simulink model "new_non_linear"  (R2022b)
settings: Solver=VariableStepAuto  StartTime=0.0  StopTime=10.0  RelTol=1e-3
values from neighbouring files (symbols this model uses):
  e_AG = 0.2    [constantes_NoLineal.m]
  e_AN = 0.2    [constantes_NoLineal.m]
  e_GA = 1-e_AG    (= 0.8)    [constantes_NoLineal.m]
  e_GP = 0.7    [constantes_NoLineal.m]
  e_NA = 1-e_AN    (= 0.8)    [constantes_NoLineal.m]
  e_NP = 0.7    [constantes_NoLineal.m]
  pob_a = 50000    [constantes_NoLineal.m]
  pob_g = 30000    [constantes_NoLineal.m]
  pob_n = 30000    [constantes_NoLineal.m]
  pob_p = 50000    [constantes_NoLineal.m]
  rc_a = 0.003    [constantes_NoLineal.m]
  rc_g = 0.8    [constantes_NoLineal.m]
  rc_n = 0.8    [constantes_NoLineal.m]
  rc_p = 0.003    [constantes_NoLineal.m]
  scale = 1    [constantes_NoLineal.m]
  T_a = 0.2    [constantes_NoLineal.m]
  T_g = 0.7    [constantes_NoLineal.m]
  T_n = 0.7    [constantes_NoLineal.m]
  T_p = 0.2    [constantes_NoLineal.m]
settings Model: Creator=mluser  LastModifiedBy=Hoyos O

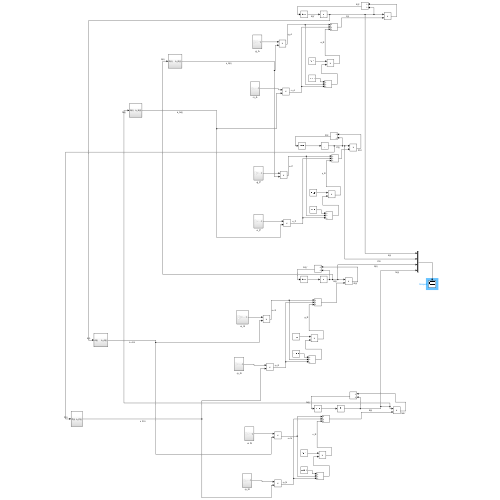
[thumbnail: Simulink's stored preview of the top-level diagram]
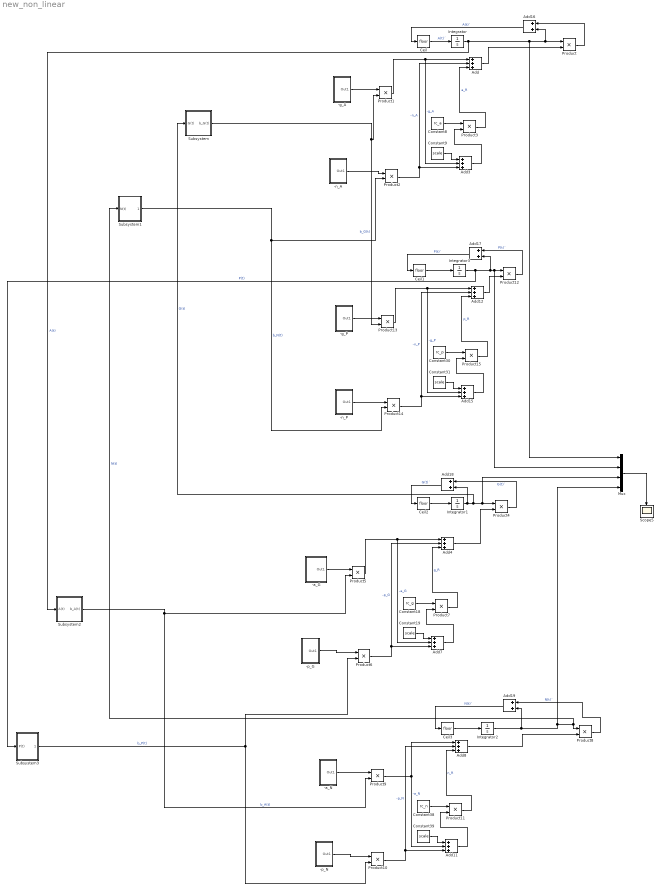
== system new_non_linear ==
  -a_G : Subsystem
  -a_N : Subsystem
  -g_A : Subsystem
  -g_P : Subsystem
  -n_A : Subsystem
  -n_P : Subsystem
  -p_G : Subsystem
  -p_N : Subsystem
  Add{,3..4,7..8,11..12,15} (8 alike) : Sum  Inputs=+++
  Add{16..19} (4 alike) : Sum
  Ceil{,1..3} (4 alike) : Rounding
  Constant18 : Constant  Value=rc_g
  Constant{9,19,31,39} (4 alike) : Constant  Value=scale
  Constant30 : Constant  Value=rc_p
  Constant38 : Constant  Value=rc_n
  Constant8 : Constant  Value=rc_a
  Integrator : Integrator  InitialCondition=pob_a
  Integrator1 : Integrator  InitialCondition=pob_g
  Integrator2 : Integrator  InitialCondition=pob_n
  Integrator3 : Integrator  InitialCondition=pob_p
  Mux : Mux
  Product{,1..15} (16 alike) : Product
  Scope5 : Scope
  Subsystem : Subsystem
  Subsystem1 : Subsystem
  Subsystem2 : Subsystem
  Subsystem3 : Subsystem
  wires:
  Integrator/1 -> Subsystem2/1(A(t)), Mux/1, Add16/2, Product/1  "A(t)"
  Add/1 -> Product/2
  Product1/1 -> Add3/2, Add/1  "-g_A"
  Product2/1 -> Add3/3, Add/2  "-n_A"
  Product3/1 -> Add/3  "a_R"
  Add3/1 -> Product3/2
  Constant8/1 -> Product3/1
  Constant9/1 -> Add3/1
  Add16/1 -> Ceil/1  "A(t)´"
  Add7/1 -> Product7/2
  Add4/1 -> Product4/2
  Integrator1/1 -> Add18/2, Subsystem/1(G(t)), Mux/3, Product4/1  "G(t)"
  Add18/1 -> Ceil2/1  "G(t)´"
  Constant19/1 -> Add7/1
  Constant18/1 -> Product7/1
  Product7/1 -> Add4/3  "g_R"
  Product6/1 -> Add7/3, Add4/2  "-p_G"
  Product5/1 -> Add7/2, Add4/1  "-a_G"
  Add15/1 -> Product15/2
  Add11/1 -> Product11/2
  Add17/1 -> Ceil1/1  "P(t)´"
  Constant31/1 -> Add15/1
  Add8/1 -> Product8/2
  Integrator2/1 -> Add19/2, Mux/4, Subsystem1/1(N(t)), Product8/1  "N(t)"
  Constant38/1 -> Product11/1
  Product11/1 -> Add8/3  "n_R"
  Product10/1 -> Add11/3, Add8/2  "-p_N"
  Product14/1 -> Add15/3, Add12/2  "-n_P"
  Constant39/1 -> Add11/1
  Integrator3/1 -> Subsystem3/1(P(t)), Add17/2, Mux/2, Product12/1  "P(t)"
  Product13/1 -> Add15/2, Add12/1  "-g_P"
  Add19/1 -> Ceil3/1  "N(t)´"
  Product9/1 -> Add8/1, Add11/2  "-a_N"
  Constant30/1 -> Product15/1
  Add12/1 -> Product12/2
  Product15/1 -> Add12/3  "p_R"
  Mux/1 -> Scope5/1
  Ceil/1 -> Integrator/1  "A(t)´"
  Ceil1/1 -> Integrator3/1
  Ceil2/1 -> Integrator1/1
  Ceil3/1 -> Integrator2/1
  Product/1 -> Add16/1
  Product12/1 -> Add17/1  "P(t)´"
  Product4/1 -> Add18/1  "G(t)´"
  Product8/1 -> Add19/1  "N(t)´"
  -a_N/1(Out1) -> Product9/1
  Subsystem/1(b_G(t)) -> Product13/2, Product1/2  "b_G(t)"
  Subsystem1/1(b_N(t)) -> Product2/2, Product14/2  "b_N(t)"
  Subsystem2/1(b_A(t)) -> Product5/2, Product9/2  "b_A(t)"
  Subsystem3/1(b_P(t)) -> Product6/2, Product10/2  "b_P(t)"
  -p_N/1(Out1) -> Product10/1
  -p_G/1(Out1) -> Product6/1
  -a_G/1(Out1) -> Product5/1
  -n_P/1(Out1) -> Product14/1
  -g_P/1(Out1) -> Product13/1
  -n_A/1(Out1) -> Product2/1
  -g_A/1(Out1) -> Product1/1

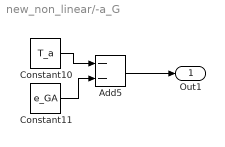
== system new_non_linear/-a_G ==
  Add5 : Sum  Inputs=--
  Constant10 : Constant  Value=T_a
  Constant11 : Constant  Value=e_GA
  Out1 : Outport
  wires:
  Constant11/1 -> Add5/2
  Constant10/1 -> Add5/1
  Add5/1 -> Out1/1

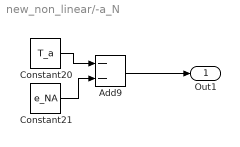
== system new_non_linear/-a_N ==
  Add9 : Sum  Inputs=--
  Constant20 : Constant  Value=T_a
  Constant21 : Constant  Value=e_NA
  Out1 : Outport
  wires:
  Constant21/1 -> Add9/2
  Constant20/1 -> Add9/1
  Add9/1 -> Out1/1

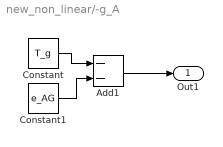
== system new_non_linear/-g_A ==
  Add1 : Sum  Inputs=--
  Constant : Constant  Value=T_g
  Constant1 : Constant  Value=e_AG
  Out1 : Outport
  wires:
  Constant/1 -> Add1/1
  Constant1/1 -> Add1/2
  Add1/1 -> Out1/1

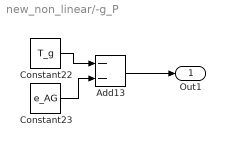
== system new_non_linear/-g_P ==
  Add13 : Sum  Inputs=--
  Constant22 : Constant  Value=T_g
  Constant23 : Constant  Value=e_AG
  Out1 : Outport
  wires:
  Constant22/1 -> Add13/1
  Constant23/1 -> Add13/2
  Add13/1 -> Out1/1

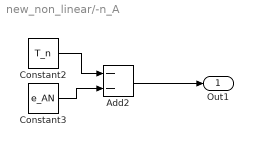
== system new_non_linear/-n_A ==
  Add2 : Sum  Inputs=--
  Constant2 : Constant  Value=T_n
  Constant3 : Constant  Value=e_AN
  Out1 : Outport
  wires:
  Constant3/1 -> Add2/2
  Constant2/1 -> Add2/1
  Add2/1 -> Out1/1

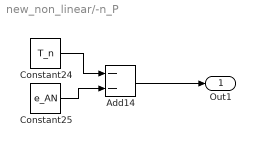
== system new_non_linear/-n_P ==
  Add14 : Sum  Inputs=--
  Constant24 : Constant  Value=T_n
  Constant25 : Constant  Value=e_AN
  Out1 : Outport
  wires:
  Constant25/1 -> Add14/2
  Constant24/1 -> Add14/1
  Add14/1 -> Out1/1

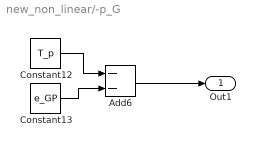
== system new_non_linear/-p_G ==
  Add6 : Sum  Inputs=--
  Constant12 : Constant  Value=T_p
  Constant13 : Constant  Value=e_GP
  Out1 : Outport
  wires:
  Constant13/1 -> Add6/2
  Add6/1 -> Out1/1
  Constant12/1 -> Add6/1

== system new_non_linear/-p_N ==
  Add10 : Sum  Inputs=--
  Constant32 : Constant  Value=T_p
  Constant33 : Constant  Value=e_NP
  Out1 : Outport
  wires:
  Constant33/1 -> Add10/2
  Add10/1 -> Out1/1
  Constant32/1 -> Add10/1

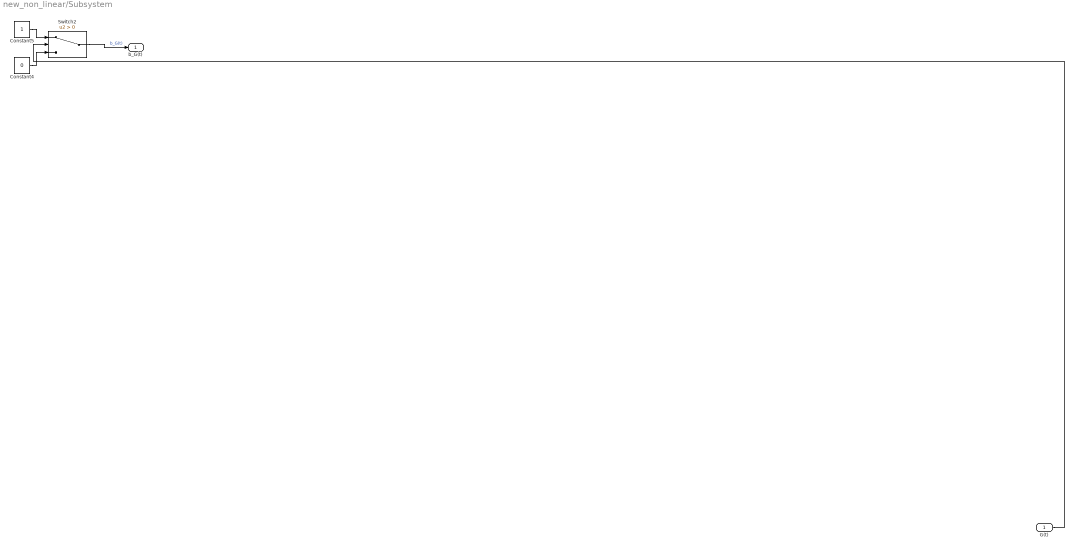
== system new_non_linear/Subsystem ==
  G(t) : Inport
  Constant4 : Constant  Value=0
  Constant5 : Constant
  Switch2 : Switch  Criteria=u2 > Threshold  SaturateOnIntegerOverflow=off  InputSameDT=off
  b_G(t) : Outport
  wires:
  Constant4/1 -> Switch2/3
  Switch2/1 -> b_G(t)/1  "b_G(t)"
  G(t)/1 -> Switch2/2
  Constant5/1 -> Switch2/1

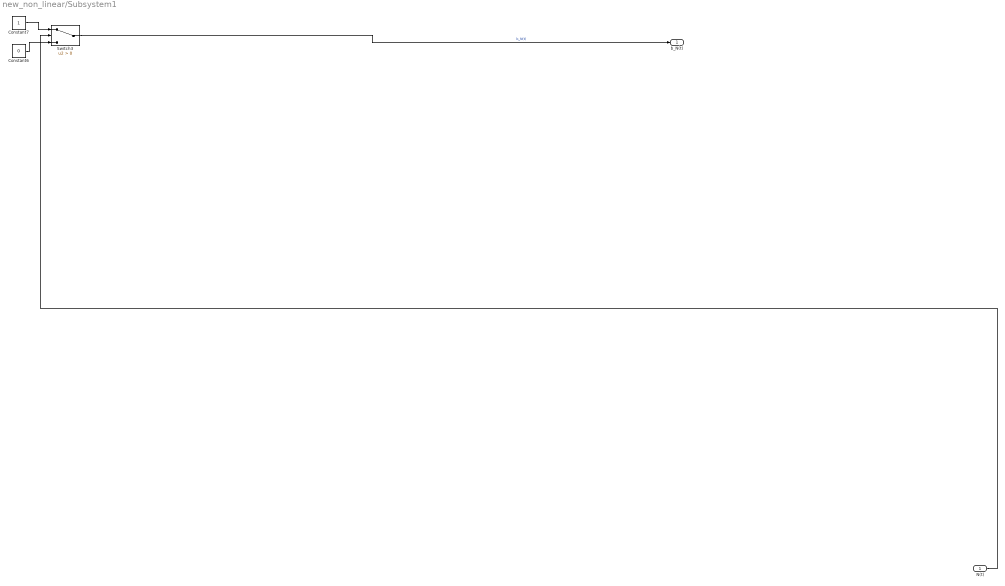
== system new_non_linear/Subsystem1 ==
  N(t) : Inport
  Constant6 : Constant  Value=0
  Constant7 : Constant
  Switch3 : Switch  Criteria=u2 > Threshold  SaturateOnIntegerOverflow=off  InputSameDT=off
  b_N(t) : Outport
  wires:
  Constant7/1 -> Switch3/1
  Constant6/1 -> Switch3/3
  Switch3/1 -> b_N(t)/1  "b_N(t)"
  N(t)/1 -> Switch3/2

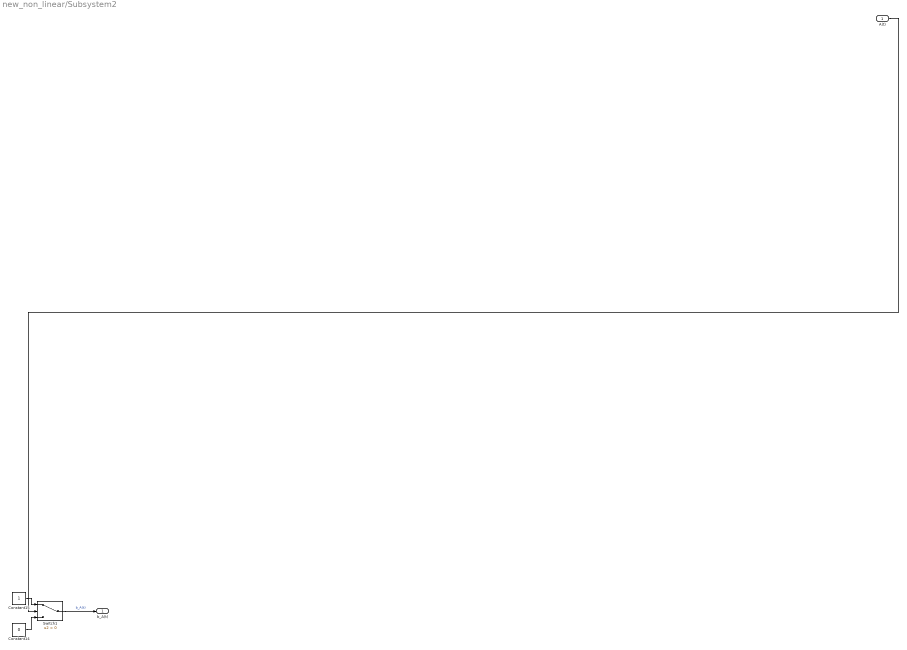
== system new_non_linear/Subsystem2 ==
  A(t) : Inport
  Constant14 : Constant  Value=0
  Constant15 : Constant
  Switch1 : Switch  Criteria=u2 > Threshold  SaturateOnIntegerOverflow=off  InputSameDT=off
  b_A(t) : Outport
  wires:
  Constant15/1 -> Switch1/1
  Constant14/1 -> Switch1/3
  A(t)/1 -> Switch1/2
  Switch1/1 -> b_A(t)/1  "b_A(t)"

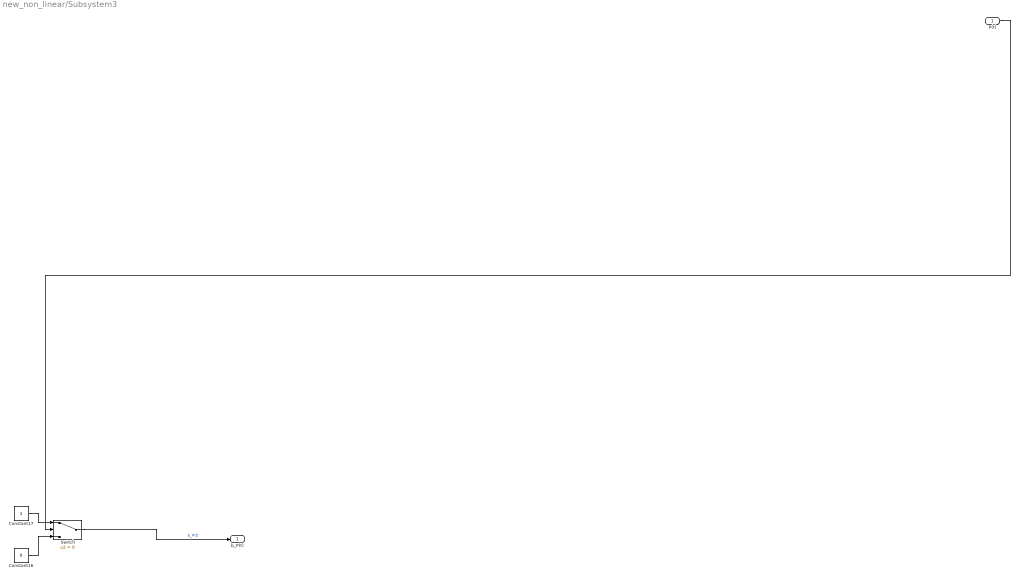
== system new_non_linear/Subsystem3 ==
  P(t) : Inport
  Constant16 : Constant  Value=0
  Constant17 : Constant
  Switch : Switch  Criteria=u2 > Threshold  SaturateOnIntegerOverflow=off  InputSameDT=off
  b_P(t) : Outport
  wires:
  Constant16/1 -> Switch/3
  Constant17/1 -> Switch/1
  P(t)/1 -> Switch/2
  Switch/1 -> b_P(t)/1  "b_P(t)"
